simulink model "fullbridge_inverter_emi"  (R2019b)
settings: Solver=VariableStepAuto  StartTime=0.0  StopTime=0.1  RelTol=1e-3
libraries: powerlib x14, dsparch4 x2, dspxfrm3 x1, dspfdesign x1, powerlib_meascontrol x1
settings Model: Creator=DELL  LastModifiedBy=DELL

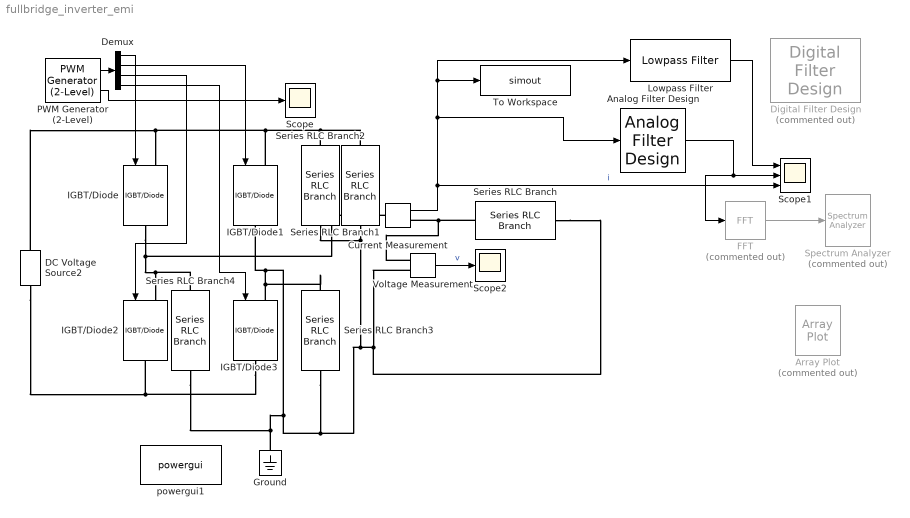
== system fullbridge_inverter_emi ==
  Analog Filter Design : dsparch4/Analog Filter Design  method=Chebyshev I  filttype=Lowpass  N=2  Wlo=400  Whi=80  Rp=3  Rs=40
  Array Plot : ArrayPlot  Commented=on
  Current Measurement : powerlib/Measurements/Current Measurement  PhasorSimulation=off  OutputType=Complex  PSBequivalent=0
      settings: SourceProductName=Simscape Electrical
  DC Voltage Source2 : powerlib/Electrical Sources/DC Voltage Source  Amplitude=400  Measurements=None
      settings: SourceProductName=Simscape Electrical
  Demux : Demux
  Digital Filter Design : dsparch4/Digital Filter Design  Commented=on  mwdsp_browser_bugfix_var=off
  FFT : dspxfrm3/FFT  Commented=on  FFTImplementation=Auto  CompMethod=Table lookup  TableOpt=NEW  TableOptActive=Speed  BitRevOrder=off  Normalize=on  InheritFFTLength=off  FFTLength=64  WrapInput=on  roundingMode=Floor  overflowMode=off  firstCoeffDataTypeStr=Inherit: Same word length as input  firstCoeffLastDataTypeStr=Inherit: Same word length as input  outputMin=[]  outputMax=[]
  Ground : powerlib/Elements/Ground  LConnTagsString=a
      settings: SourceProductName=Simscape Electrical
  IGBT/Diode{,1..3} (4 alike) : powerlib/Power Electronics/IGBT//Diode  Ron=1e-3  Rs=1e5  Cs=inf  Measurements=off
      settings: SourceProductName=Simscape Electrical
  Lowpass Filter : dspfdesign/Lowpass Filter  FilterType=IIR  DesignForMinimumOrder=on  FilterOrder=50  PassbandFrequency=60  StopbandFrequency=140  PassbandRipple=0.1  StopbandAttenuation=23  InheritSampleRate=on  SampleRate=44100  SimulateUsing=Interpreted execution  roundingMode=Floor  coeffsDataTypeStr=fixdt(1,16)
  PWM Generator (2-Level) : powerlib_meascontrol/Pulse & Signal Generators/PWM Generator (2-Level)  ModulatorType=Single-phase full-bridge (4 pulses)  ModulatorMode=Unsynchronized  Fc=27*60  Pc=90  nF=27  MinMax="[ -1  1 ]"  SamplingTechnique=Natural  ModulatingSignals=on  m=0.8  Freq=50  Phase=0  Ts=5e-7  ShowCarrierOutport=on
  Scope : Scope
  Scope1 : Scope  NumInputPorts=3
  Scope2 : Scope
  Series RLC Branch : powerlib/Elements/Series RLC Branch  LConnTagsString=__new0  RConnTagsString=__new0  BranchType=RL  Resistance=1  Inductance=5e-3  SetiL0=off  InitialCurrent=0  Capacitance=1e-6  Setx0=off  InitialVoltage=0  Measurements=None
      settings: SourceProductName=Simscape Electrical
  Series RLC Branch{1..4} (4 alike) : powerlib/Elements/Series RLC Branch  LConnTagsString=__new0  RConnTagsString=__new0  BranchType=C  Resistance=2.9  Inductance=1e-3  SetiL0=off  InitialCurrent=0  Capacitance=2e-8  Setx0=off  InitialVoltage=0  Measurements=None
      settings: SourceProductName=Simscape Electrical
  Spectrum Analyzer : SpectrumAnalyzer  Commented=on
  To Workspace : ToWorkspace  VariableName=simout  SaveFormat=Timeseries  SampleTime=-1
  Voltage Measurement : powerlib/Measurements/Voltage Measurement  PhasorSimulation=off  OutputType=Complex  PSBequivalent=0
      settings: SourceProductName=Simscape Electrical
  powergui1 : powerlib/powergui  Priority=1  SimulationMode=Discrete  SampleTime=5e-7  frequency=60  Iterations=50  frequencyindice=0  Pbase=100e6  ErrMax=1e-4  UnitsV=kV  UnitsW=MW  buscounter=0  FunctionMessages=off  echomessages=off  EnableUseOfTLC=off  CurrentSourceSwitches=off  DisableSnubberDevices=off  DisableRonSwitches=off  DisableVfSwitches=off  DisplayEquations=off  AutomaticDiscreteSolvers=off  SolverType=Tustin/Backward Euler (TBE)  Interpol=off  ExternalGateDelay=off  methode=off  Ts=100  x0status=blocks  SPID=on  SwTol=0  HookPort=off  NonlinearTolerance=1e-4  nMaxIteration=100  ContinueOnMaxIteration=off  RestoreLinks=warning  ResistiveCurrentMeasurement=off  Frange=[0:2:500]  Ylog=off  Xlog=on  ShowGrid=off  save=off  variable=ZData  structure=0  ZoomFFT=off  StartTime=0.0  cycles=1  DisplayStyle=1  fundamental=60  FreqAxis=off  MaxFrequency=1000  frequencyindicesteady=1  RmsSteady=1  display=off
      settings: SourceProductName=Simscape Electrical
  wires:
  PWM Generator (2-Level)/1 -> Demux/1
  Demux/1 -> IGBT/Diode/1
  Demux/2 -> IGBT/Diode1/1
  Demux/3 -> IGBT/Diode2/1
  Demux/4 -> IGBT/Diode3/1
  Current Measurement/1 -> Analog Filter Design/1, Lowpass Filter/1, To Workspace/1, Scope1/3  "i"
  Voltage Measurement/1 -> Scope2/1  "v"
  PWM Generator (2-Level)/2 -> Scope/1
  Analog Filter Design/1 -> FFT/1, Scope1/2
  Lowpass Filter/1 -> Scope1/1
  FFT/1 -> Spectrum Analyzer/1
  connections:
  IGBT/Diode3/LConn1 -- Series RLC Branch3/LConn1 -- Series RLC Branch4/RConn1 -- Ground/LConn1 -- Series RLC Branch3/RConn1 -- Series RLC Branch2/RConn1 -- Series RLC Branch1/RConn1 -- Voltage Measurement/LConn2 -- Series RLC Branch/RConn1 -- IGBT/Diode1/RConn1
  Series RLC Branch/LConn1 -- Voltage Measurement/LConn1 -- Current Measurement/RConn1
  IGBT/Diode3/RConn1 -- DC Voltage Source2/LConn1 -- IGBT/Diode2/RConn1
  DC Voltage Source2/RConn1 -- Series RLC Branch1/LConn1 -- Series RLC Branch2/LConn1 -- IGBT/Diode1/LConn1 -- IGBT/Diode/LConn1
  IGBT/Diode/RConn1 -- Current Measurement/LConn1 -- Series RLC Branch4/LConn1 -- IGBT/Diode2/LConn1
